simulink model "daixianPAM_11"  (R2018a)
settings: Solver=VariableStepAuto  StartTime=0.0  StopTime=10.0  RelTol=1e-3
libraries: commutil2 x4, commsink2 x2, commdigbbndam3 x2, commfilt2 x2, commchan3 x1, commrandsrc3 x1
settings Model: Creator=sdf  LastModifiedBy=sdf

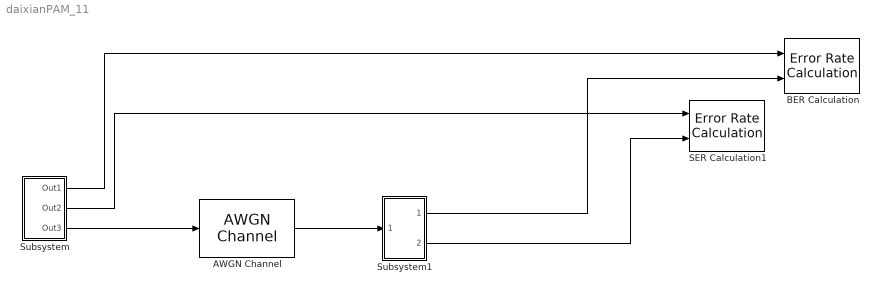
== system daixianPAM_11 ==
  AWGN Channel : commchan3/AWGN Channel  InputProcessing=Columns as channels (frame based)  seed=1234  noiseMode="Signal to noise ratio  (Es/No)"  EbNodB=10  EsNodB=SNR  SNRdB=10  bitsPerSym=1  Ps=5  Tsym=1/100000  variance=1
  BER Calculation : commsink2/Error Rate Calculation  N=0  st_delay=0  cp_mode=Entire frame  subframe=[]  PMode=Workspace  WsName=BER  RsMode2=off  stop=off  numErr=100  maxBits=1e6
  SER Calculation1 : commsink2/Error Rate Calculation  N=0  st_delay=0  cp_mode=Entire frame  subframe=[]  PMode=Workspace  WsName=SER  RsMode2=off  stop=off  numErr=100  maxBits=1e6
  Subsystem : Subsystem
  Subsystem1 : Subsystem
  wires:
  Subsystem/1(Out1) -> BER Calculation/1
  Subsystem/2(Out2) -> SER Calculation1/1
  Subsystem/3(Out3) -> AWGN Channel/1
  AWGN Channel/1 -> Subsystem1/1(In1)
  Subsystem1/1(Out1) -> BER Calculation/2
  Subsystem1/2(Out2) -> SER Calculation1/2

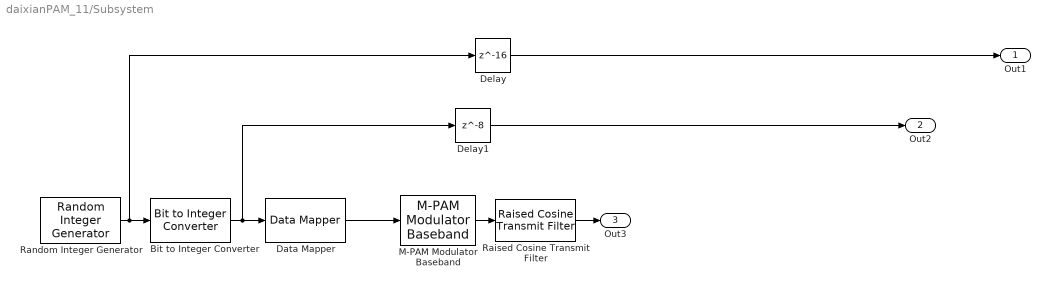
== system daixianPAM_11/Subsystem ==
  Bit to Integer Converter : commutil2/Bit to Integer Converter  nbits=2  bitOrder=MSB first  signedOutputValues=Unsigned  outDtype=Inherit via internal rule  outDtypeSigned=Inherit via internal rule
  Data Mapper : commutil2/Data Mapper  MapMode=Binary to Gray  M=4  MapVec=[0 1 3 2 7 6 4 5]
      settings: SourceProductName=Communications System Toolbox  SourceProductBaseCode=CM
  Delay : Delay  DelayLength=16  InitialCondition=0
  Delay1 : Delay  DelayLength=8  InitialCondition=0
  M-PAM Modulator Baseband : commdigbbndam3/M-PAM Modulator Baseband  M=4  InType=Integer  Enc=Binary  PowType=Min. distance between symbols  MinDist=2  AvgPow=1  PeakPow=1  outDtype=double  outWordLen=16  outUDDataType=sfix(16)  outFracLenMode=Best precision  outFracLen=15  outDataTypeStr=double  outLastDataTypeStr=double
      settings: SourceProductName=Communications System Toolbox  SourceProductBaseCode=CM
  Raised Cosine Transmit Filter : commfilt2/Raised Cosine Transmit Filter  filtType=Square root  R=0.25  filtSpan=4  N=10  filterGain=1  InputProcessing=Columns as channels (frame based)  RateOptions=Enforce single-rate processing  framing=Mute  checkCoeff=off  variableName=rcTxFilt  checkGain=Normalized  sampMode=Mute  saveAsFlag=0  currentFiltSpan=4  D=(4)/2  launchFVT=on  roundingMode=Floor  overflowMode=off  coeffDataTypeStr=Inherit: Same word length as input  coeffMin=[]  coeffMax=[]  coeffLastDataTypeStr=Inherit: Same word length as input  outputDataTypeStr=Inherit: Same as accumulator  outputMin=[]  outputMax=[]  outputLastDataTypeStr=Inherit: Same as accumulator
  Random Integer Generator : commrandsrc3/Random Integer Generator  SetSize=2  SeedSource=Auto  Seed=0  SampleTime=1/200000  SamplesPerFrame=20000  OutputDataType=double  SimulateUsing=Interpreted execution
  Out1 : Outport
  Out2 : Outport  Port=2
  Out3 : Outport  Port=3
  wires:
  Data Mapper/1 -> M-PAM Modulator Baseband/1
  Bit to Integer Converter/1 -> Delay1/1, Data Mapper/1
  Random Integer Generator/1 -> Delay/1, Bit to Integer Converter/1
  M-PAM Modulator Baseband/1 -> Raised Cosine Transmit Filter/1
  Raised Cosine Transmit Filter/1 -> Out3/1
  Delay1/1 -> Out2/1
  Delay/1 -> Out1/1

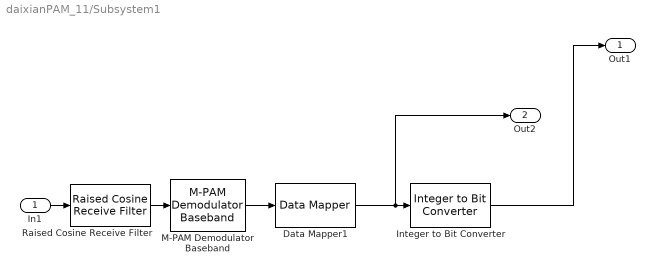
== system daixianPAM_11/Subsystem1 ==
  In1 : Inport
  Data Mapper1 : commutil2/Data Mapper  MapMode=Binary to Gray  M=4  MapVec=[0 1 3 2 7 6 4 5]
      settings: SourceProductName=Communications System Toolbox  SourceProductBaseCode=CM
  Integer to Bit Converter : commutil2/Integer to Bit Converter  nbits=2  signedInputValues=Unsigned  bitOrder=MSB first  outDtype=Inherit via internal rule
  M-PAM Demodulator Baseband : commdigbbndam3/M-PAM Demodulator Baseband  M=4  OutType=Integer  Dec=Binary  PowType=Min. distance between symbols  MinDist=2  AvgPow=1  PeakPow=1  outDtype1=Inherit via internal rule  outDtype2=Inherit via internal rule  denormFactorWordLen=16  denormFactorDataTypeStr=Inherit: Same word length as input  denormFactorLastDataTypeStr=Inherit: Same word length as input  prodOutWordLen=16  prodOutRoundingMode=Floor  prodOutOverflowMode=Wrap  prodOutOvFlMode=off  prodOutOvFlModeLastStrValue=off  sumWordLen=16
      settings: SourceProductName=Communications System Toolbox  SourceProductBaseCode=CM
  Raised Cosine Receive Filter : commfilt2/Raised Cosine Receive Filter  filtType=Square root  R=0.25  filtSpan=4  N=10  downFactor=10  downOffset=0  filterGain=1  InputProcessing=Columns as channels (frame based)  RateOptions=Enforce single-rate processing  framing=Mute  checkCoeff=off  variableName=rcRxFilt  currentFiltSpan=4  D=(4)/2  inputOffset=0  sampMode=Mute  saveAsFlag=0  rateMode=Downsampling  checkGain=Normalized  launchFVT=on  roundingMode=Floor  overflowMode=off  coeffDataTypeStr=Inherit: Same word length as input  coeffMin=[]  coeffMax=[]  coeffLastDataTypeStr=Inherit: Same word length as input  accumDataTypeStr=Inherit: Same as product output  accumLastDataTypeStr=Inherit: Same as product output  outputDataTypeStr=Inherit: Same as accumulator  outputMin=[]  outputMax=[]  outputLastDataTypeStr=Inherit: Same as accumulator
  Out1 : Outport
  Out2 : Outport  Port=2
  wires:
  Integer to Bit Converter/1 -> Out1/1
  In1/1 -> Raised Cosine Receive Filter/1
  M-PAM Demodulator Baseband/1 -> Data Mapper1/1
  Data Mapper1/1 -> Out2/1, Integer to Bit Converter/1
  Raised Cosine Receive Filter/1 -> M-PAM Demodulator Baseband/1
